simulink model "induction_machine"  (R2012b)
settings: Solver=ode23s  StartTime=0.0  StopTime=1.0  MaxStep=2e-5  RelTol=1e-5
undefined symbols (not defined in the file or in its folder): j
libraries: powerlib x12
settings Model: Creator=Pietro  LastModifiedBy=Pietro
settings SolverCC: ZeroCrossControl=DisableAll
settings DataIOCC: SignalLoggingSaveFormat=ModelDataLogs
settings OptimizationCC: InlineInvariantSignals=on  InitFltsAndDblsToZero=on
settings DebuggingCC: SaveWithParameterizedLinksMsg=none  SignalResolutionControl=TryResolveAllWithWarning  MultiTaskDSMMsg=warning  MultiTaskCondExecSysMsg=none  FcnCallInpInsideContextMsg=UseLocalSettings  StrictBusMsg=None
settings RTWCC: IncludeERTFirstTime=on
settings GRTTargetCC: TargetFcnLib=ansi_tfl_tmw.mat  CombineOutputUpdateFcns=off  GRTInterface=on

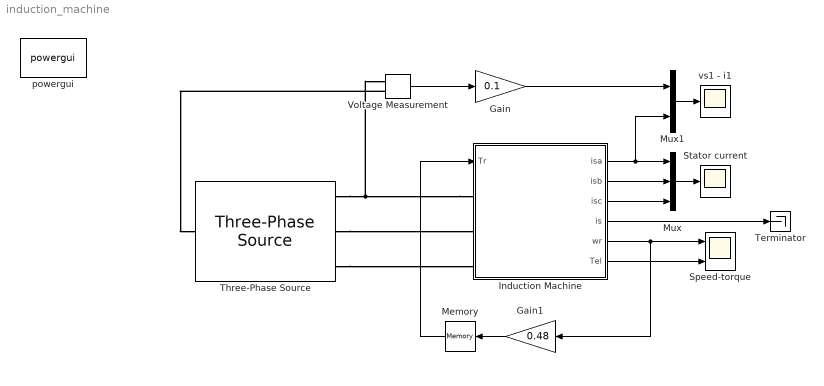
== system induction_machine ==
  Gain : Gain  Gain=0.1
  Gain1 : Gain  Gain=0.48
  Induction Machine : Subsystem  mask{ls=0.004, Lm=0.057, lr=0.004, rs=0.52, rr=0.5, p=2, J=0.23}
      mask help:
      | Inserire i parametri della macchina sincrona.
      | kecc = zs / zecc
  Memory : Memory
  Mux : Mux  Inputs=3
  Mux1 : Mux  Inputs=2
  Speed-torque : Scope  NumInputPorts=2
      settings: YMin=-25~-100  YMax=150~200  SaveName=pippo
  Stator current : Scope
      settings: YMin=-150  YMax=150
  Terminator : Terminator
  Three-Phase Source : powerlib/Electrical Sources/Three-Phase Source  Voltage=415  PhaseAngle=0  Frequency=50  InternalConnection=Yn  SpecifyImpedance=on  Resistance=0.8929  Inductance=16.58e-3  ShortCircuitLevel=1000e3  BaseVoltage=400  XRratio=7  BusType=swing  Pref=0  Qref=0  Qmin=-inf  Qmax=inf
  Voltage Measurement : powerlib/Measurements/Voltage Measurement  PhasorSimulation=off  OutputType=Complex  PSBequivalent=0
  powergui : powerlib/powergui  Priority=1  SimulationMode=Continuous  SolverType=Tustin  SampleTime=50e-6  frequency=60  SPID=off  DisableSnubberDevices=off  DisableRonSwitches=off  DisableVfSwitches=off  SwTol=0  Interpol=off  DisplayEquations=off  FunctionMessages=off  frequencyindice=50  Pbase=100e6  ErrMax=1e-4  Iterations=50  UnitsV=kV  UnitsW=MW  echomessages=off  HookPort=off  EnableUseOfTLC=off  x0status=blocks  RestoreLinks=warning  ResistiveCurrentMeasurement=off  Ylog=off  Xlog=on  ShowGrid=off  save=off  variable=ZData  ZoomFFT=off  StartTime=0.0  cycles=1  DisplayStyle=1  FreqAxis=off  MaxFrequency=1000  frequencyindicesteady=1  display=off  methode=off
  vs1 - i1 : Scope
      settings: YMin=-225  YMax=150  SaveName=ScopeData3
  wires:
  Induction Machine/1(isa) -> Mux/1, Mux1/2
  Induction Machine/2(isb) -> Mux/2
  Induction Machine/3(isc) -> Mux/3
  Mux/1 -> Stator current/1
  Voltage Measurement/1 -> Gain/1
  Mux1/1 -> vs1 - i1/1
  Gain/1 -> Mux1/1
  Induction Machine/5(wr) -> Gain1/1, Speed-torque/1
  Induction Machine/6(Tel) -> Speed-torque/2
  Gain1/1 -> Memory/1
  Induction Machine/4(is) -> Terminator/1
  Memory/1 -> Induction Machine/1(Tr)
  connections:
  Three-Phase Source/RConn2 -- Induction Machine/LConn2
  Three-Phase Source/RConn3 -- Induction Machine/LConn3
  Voltage Measurement/LConn2 -- Three-Phase Source/LConn1
  Induction Machine/LConn1 -- Three-Phase Source/RConn1 -- Voltage Measurement/LConn1

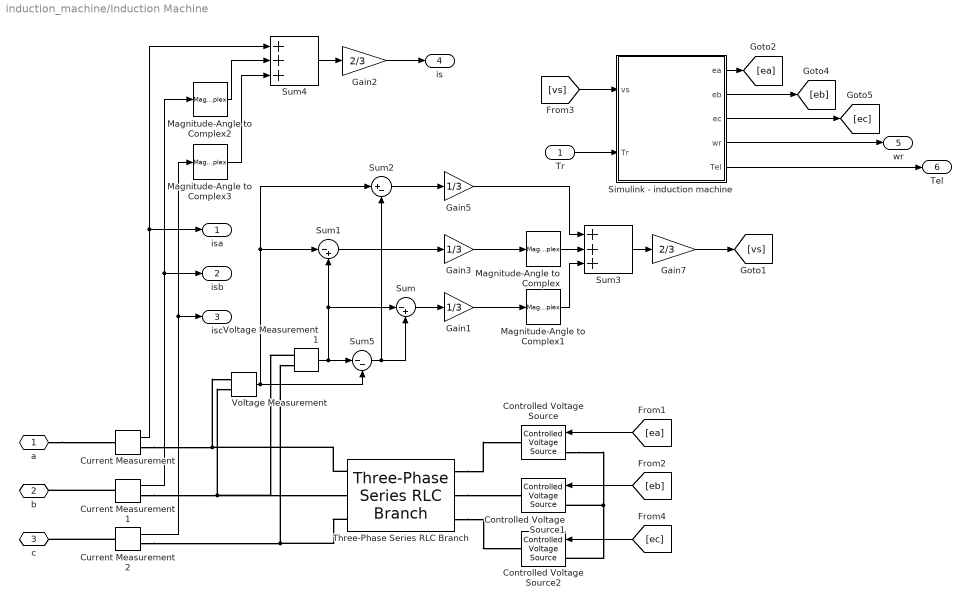
== system induction_machine/Induction Machine ==
  Tr : Inport
  Controlled Voltage Source : powerlib/Electrical Sources/Controlled Voltage Source  Initialize=off  Source_Type=AC  Amplitude=0  Phase=0  Frequency=0  Measurements=None
  Controlled Voltage Source1 : powerlib/Electrical Sources/Controlled Voltage Source  Initialize=off  Source_Type=AC  Amplitude=0  Phase=0  Frequency=0  Measurements=None
  Controlled Voltage Source2 : powerlib/Electrical Sources/Controlled Voltage Source  Initialize=off  Source_Type=AC  Amplitude=0  Phase=0  Frequency=0  Measurements=None
  Current Measurement : powerlib/Measurements/Current Measurement  PhasorSimulation=off  OutputType=Complex  PSBequivalent=0
  Current Measurement1 : powerlib/Measurements/Current Measurement  PhasorSimulation=off  OutputType=Complex  PSBequivalent=0
  Current Measurement2 : powerlib/Measurements/Current Measurement  PhasorSimulation=off  OutputType=Complex  PSBequivalent=0
  Gain1 : Gain  Gain=1/3
  Gain2 : Gain  Gain=2/3
  Gain3 : Gain  Gain=1/3
  Gain5 : Gain  Gain=1/3
  Gain7 : Gain  Gain=2/3
  Magnitude-Angle to Complex : MagnitudeAngleToComplex  Input=Magnitude  ConstantPart=2*pi/3
  Magnitude-Angle to Complex1 : MagnitudeAngleToComplex  Input=Magnitude  ConstantPart=4*pi/3
  Magnitude-Angle to Complex2 : MagnitudeAngleToComplex  Input=Magnitude  ConstantPart=2*pi/3
  Magnitude-Angle to Complex3 : MagnitudeAngleToComplex  Input=Magnitude  ConstantPart=4*pi/3
  Simulink - induction machine : Subsystem
  Sum : Sum  Inputs=|-+
  Sum1 : Sum  Inputs=|-+
  Sum2 : Sum  Inputs=|+-
  Sum3 : Sum  Inputs=+++
  Sum4 : Sum  Inputs=+++
  Sum5 : Sum  Inputs=|--
  Three-Phase Series RLC Branch : powerlib/Elements/Three-Phase Series RLC Branch  LConnTagsString=A|B|C  RConnTagsString=A|B|C  BranchType=RL  Resistance=rs  Inductance=ls  Capacitance=[]  Measurements=None
  Voltage Measurement : powerlib/Measurements/Voltage Measurement  PhasorSimulation=off  OutputType=Complex  PSBequivalent=0
  Voltage Measurement1 : powerlib/Measurements/Voltage Measurement  PhasorSimulation=off  OutputType=Complex  PSBequivalent=0
  a : PMIOPort  Port=1  Side=Left
  b : PMIOPort  Port=2  Side=Left
  c : PMIOPort  Port=3  Side=Left
  isa : Outport
  isb : Outport  Port=2
  isc : Outport  Port=3
  is : Outport  Port=4
  wr : Outport  Port=5
  Tel : Outport  Port=6
  wires:
  Voltage Measurement/1 -> Sum5/2, Sum1/1, Sum2/1
  Voltage Measurement1/1 -> Sum5/1, Sum1/2, Sum/1
  Sum/1 -> Gain1/1
  Sum1/1 -> Gain3/1
  Sum5/1 -> Sum2/2, Sum/2
  Sum2/1 -> Gain5/1
  Gain5/1 -> Sum3/1
  Gain3/1 -> Magnitude-Angle to Complex/1
  Gain1/1 -> Magnitude-Angle to Complex1/1
  Sum3/1 -> Gain7/1
  Magnitude-Angle to Complex/1 -> Sum3/2
  Magnitude-Angle to Complex1/1 -> Sum3/3
  Tr/1 -> Simulink - induction machine/2(Tr)
  [ea] -> Controlled Voltage Source/1
  [eb] -> Controlled Voltage Source1/1
  [ec] -> Controlled Voltage Source2/1
  Current Measurement2/1 -> isc/1, Magnitude-Angle to Complex3/1
  Current Measurement1/1 -> isb/1, Magnitude-Angle to Complex2/1
  Current Measurement/1 -> isa/1, Sum4/1
  Magnitude-Angle to Complex3/1 -> Sum4/3
  Magnitude-Angle to Complex2/1 -> Sum4/2
  Gain2/1 -> is/1
  Sum4/1 -> Gain2/1
  Simulink - induction machine/1(ea) -> [ea]
  Simulink - induction machine/2(eb) -> [eb]
  Simulink - induction machine/3(ec) -> [ec]
  Simulink - induction machine/4(wr) -> wr/1
  Simulink - induction machine/5(Tel) -> Tel/1
  Gain7/1 -> [vs]
  [vs] -> Simulink - induction machine/1(vs)
  connections:
  Three-Phase Series RLC Branch/LConn1 -- Voltage Measurement/LConn1 -- Current Measurement/RConn1
  Three-Phase Series RLC Branch/LConn3 -- Voltage Measurement1/LConn2 -- Current Measurement2/RConn1
  Voltage Measurement1/LConn1 -- Three-Phase Series RLC Branch/LConn2 -- Voltage Measurement/LConn2 -- Current Measurement1/RConn1
  Three-Phase Series RLC Branch/RConn2 -- Controlled Voltage Source1/RConn1
  Three-Phase Series RLC Branch/RConn1 -- Controlled Voltage Source/RConn1
  Three-Phase Series RLC Branch/RConn3 -- Controlled Voltage Source2/RConn1
  Controlled Voltage Source/LConn1 -- Controlled Voltage Source2/LConn1 -- Controlled Voltage Source1/LConn1
  a/RConn1 -- Current Measurement/LConn1
  Current Measurement1/LConn1 -- b/RConn1
  Current Measurement2/LConn1 -- c/RConn1

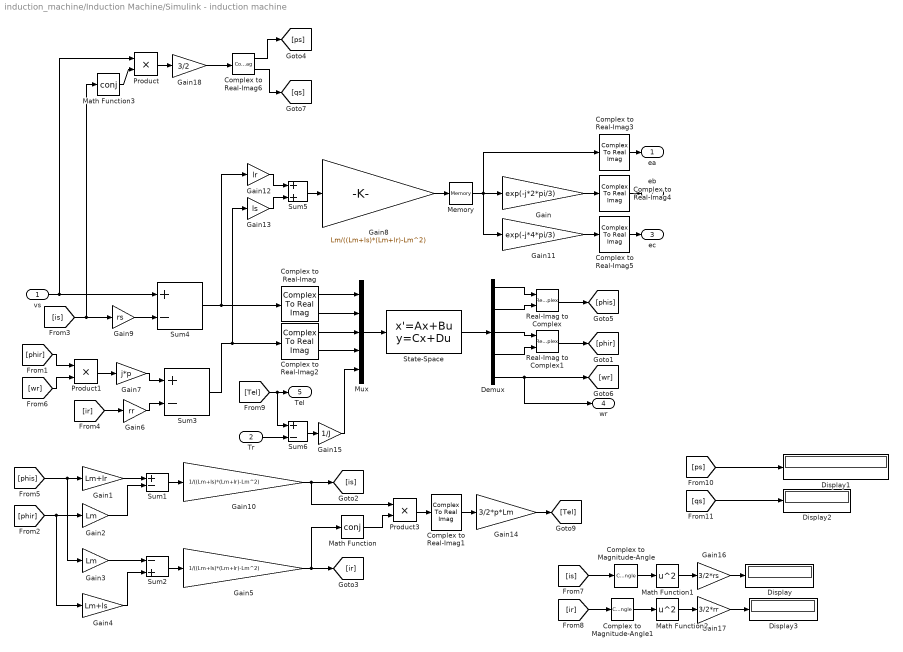
== system induction_machine/Induction Machine/Simulink - induction machine ==
  vs : Inport
  Tr : Inport  Port=2
  Complex to Magnitude-Angle : ComplexToMagnitudeAngle  Output=Magnitude
  Complex to Magnitude-Angle1 : ComplexToMagnitudeAngle  Output=Magnitude
  Complex to Real-Imag : ComplexToRealImag
  Complex to Real-Imag1 : ComplexToRealImag  Output=Imag
  Complex to Real-Imag2 : ComplexToRealImag
  Complex to Real-Imag3 : ComplexToRealImag  Output=Real
  Complex to Real-Imag4 : ComplexToRealImag  Output=Real
  Complex to Real-Imag5 : ComplexToRealImag  Output=Real
  Complex to Real-Imag6 : ComplexToRealImag
  Demux : Demux  Outputs=5
  Display{,1..3} (4 alike) : Display
  Gain : Gain  Gain=exp(-j*2*pi/3)
  Gain1 : Gain  Gain=Lm+lr
  Gain10 : Gain  Gain=1/((Lm+ls)*(Lm+lr)-Lm^2)
  Gain11 : Gain  Gain=exp(-j*4*pi/3)
  Gain12 : Gain  Gain=lr
  Gain13 : Gain  Gain=ls
  Gain14 : Gain  Gain=3/2*p*Lm
  Gain15 : Gain  Gain=1/J
  Gain16 : Gain  Gain=3/2*rs
  Gain17 : Gain  Gain=3/2*rr
  Gain18 : Gain  Gain=3/2
  Gain2 : Gain  Gain=Lm
  Gain3 : Gain  Gain=Lm
  Gain4 : Gain  Gain=Lm+ls
  Gain5 : Gain  Gain=1/((Lm+ls)*(Lm+lr)-Lm^2)
  Gain6 : Gain  Gain=rr
  Gain7 : Gain  Gain=j*p
  Gain8 : Gain  Gain=Lm/((Lm+ls)*(Lm+lr)-Lm^2)
  Gain9 : Gain  Gain=rs
  Math Function : Math  Operator=conj  SaturateOnIntegerOverflow=on
  Math Function1 : Math  Operator=square  SaturateOnIntegerOverflow=on
  Math Function2 : Math  Operator=square  SaturateOnIntegerOverflow=on
  Math Function3 : Math  Operator=conj  SaturateOnIntegerOverflow=on
  Memory : Memory
  Mux : Mux  Inputs=5
  Product : Product  RndMeth=Zero
  Product1 : Product  RndMeth=Zero
  Product3 : Product  RndMeth=Zero
  Real-Imag to Complex : RealImagToComplex
  Real-Imag to Complex1 : RealImagToComplex
  State-Space : StateSpace  A=[0,0,0,0,0; 0,0,0,0,0; 0,0,0,0,0; 0,0,0,0,0; 0,0,0,0,0]  B=[1,0,0,0,0; 0,1,0,0,0; 0,0,1,0,0; 0,0,0,1,0; 0,0,0,0,1]  C=[1,0,0,0,0; 0,1,0,0,0; 0,0,1,0,0; 0,0,0,1,0; 0,0,0,0,1]  D=[0,0,0,0,0; 0,0,0,0,0; 0,0,0,0,0; 0,0,0,0,0; 0,0,0,0,0]  X0=[0,0,0,0,0]
  Sum{1,3..4,6} (4 alike) : Sum  Inputs=+-
  Sum2 : Sum  Inputs=-+
  Sum5 : Sum
  ea : Outport
  eb : Outport  Port=2
  ec : Outport  Port=3
  wr : Outport  Port=4
  Tel : Outport  Port=5
  wires:
  State-Space/1 -> Demux/1
  Mux/1 -> State-Space/1
  Demux/1 -> Real-Imag to Complex/1
  Demux/2 -> Real-Imag to Complex/2
  Real-Imag to Complex/1 -> [phis]
  Complex to Real-Imag/1 -> Mux/1
  Complex to Real-Imag/2 -> Mux/2
  Gain14/1 -> [Tel]
  Sum6/1 -> Gain15/1
  [Tel] -> Sum6/1, Tel/1
  Tr/1 -> Sum6/2
  Demux/5 -> [wr], wr/1
  Real-Imag to Complex1/1 -> [phir]
  Demux/3 -> Real-Imag to Complex1/1
  Demux/4 -> Real-Imag to Complex1/2
  Gain15/1 -> Mux/5
  [phis] -> Gain1/1, Gain3/1
  Gain1/1 -> Sum1/1
  Gain2/1 -> Sum1/2
  [phir] -> Gain2/1, Gain4/1
  Sum1/1 -> Gain10/1
  Gain3/1 -> Sum2/1
  Gain4/1 -> Sum2/2
  Sum2/1 -> Gain5/1
  [phir] -> Product1/1
  [wr] -> Product1/2
  Product1/1 -> Gain7/1
  Gain7/1 -> Sum3/1
  Gain6/1 -> Sum3/2
  Complex to Real-Imag2/1 -> Mux/3
  Complex to Real-Imag2/2 -> Mux/4
  Sum3/1 -> Complex to Real-Imag2/1, Gain13/1
  Gain10/1 -> Product3/1, [is]
  Gain5/1 -> Math Function/1, [ir]
  [ir] -> Gain6/1
  Complex to Real-Imag1/1 -> Gain14/1
  Product3/1 -> Complex to Real-Imag1/1
  Gain11/1 -> Complex to Real-Imag5/1
  Gain/1 -> Complex to Real-Imag4/1
  Complex to Real-Imag3/1 -> ea/1
  Complex to Real-Imag4/1 -> eb/1
  Complex to Real-Imag5/1 -> ec/1
  Math Function/1 -> Product3/2
  [is] -> Gain9/1, Math Function3/1
  Gain9/1 -> Sum4/2
  vs/1 -> Sum4/1, Product/1
  Sum4/1 -> Complex to Real-Imag/1, Gain12/1
  Gain8/1 -> Memory/1
  Sum5/1 -> Gain8/1
  Gain13/1 -> Sum5/2
  Gain12/1 -> Sum5/1
  [is] -> Complex to Magnitude-Angle/1
  Complex to Magnitude-Angle/1 -> Math Function1/1
  Math Function1/1 -> Gain16/1
  Gain16/1 -> Display/1
  [ir] -> Complex to Magnitude-Angle1/1
  Complex to Magnitude-Angle1/1 -> Math Function2/1
  Math Function2/1 -> Gain17/1
  Gain17/1 -> Display3/1
  [ps] -> Display1/1
  [qs] -> Display2/1
  Memory/1 -> Gain/1, Gain11/1, Complex to Real-Imag3/1
  Product/1 -> Gain18/1
  Math Function3/1 -> Product/2
  Gain18/1 -> Complex to Real-Imag6/1
  Complex to Real-Imag6/1 -> [ps]
  Complex to Real-Imag6/2 -> [qs]
